simulink model "Cont2014"  (R2014b)
settings: Solver=ode45  StartTime=0.0  StopTime=1  RelTol=1e-3
settings Model: CovModelRefEnable=off  CovSFcnEnable=on  Creator=asuS  LastModifiedBy=asuS
settings DataIOCC: SaveFormat=StructureWithTime
settings DebuggingCC: SolverPrmCheckMsg=none  FrameProcessingCompatibilityMsg=error
settings HardwareCC: ProdBitPerPointer=64  ProdLargestAtomicFloat=Float  ProdIntDivRoundTo=Zero  ProdEndianess=LittleEndian  ProdHWDeviceType=Specified
settings GRTTargetCC: GeneratePreprocessorConditionals=Use local settings

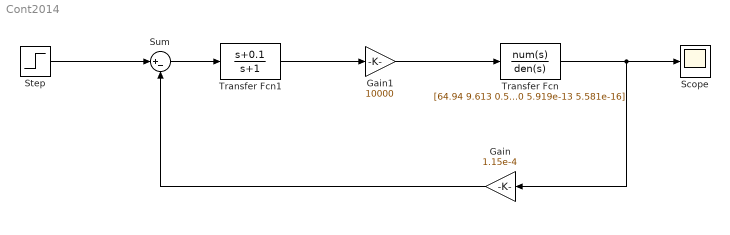
== system Cont2014 ==
  Gain : Gain  Gain=1.15e-4
  Gain1 : Gain  Gain=10000
  Scope : Scope
      settings: TimeRange=auto  MaxDataPoints=5000  SaveName=ScopeData  YMin=-0.03751  YMax=0.33762  SampleTime=-1  DataFormat=Array
  Step : Step  Time=0  After=3.4899e-5  SampleTime=0
  Sum : Sum  Inputs=|+-
  Transfer Fcn : TransferFcn  Numerator=[64.94 9.613 0.5474 0.01506 0.0002085 1.427e-6 4.358e-9 4.768e-12]  Denominator=[1 0.1595 0.009992 0.0003134 5.269e-6 4.864e-8 2.415e-10 5.919e-13 5.581e-16]
  Transfer Fcn1 : TransferFcn  Numerator=[1 0.1]  Denominator=[1 1]
  wires:
  Step/1 -> Sum/1
  Transfer Fcn/1 -> Gain/1, Scope/1
  Gain/1 -> Sum/2
  Sum/1 -> Transfer Fcn1/1
  Transfer Fcn1/1 -> Gain1/1
  Gain1/1 -> Transfer Fcn/1
